simulink model "indmot1"  (Simulink 8.5)
settings: Solver=ode45  SolverMode=SingleTasking  StartTime=0.0  StopTime=3  MaxStep=1e-3  RelTol=1e-3  AbsTol=1e-6
libraries: powerlib x26
settings Model: Creator=PC  LastModifiedBy=PC
settings DataIOCC: LimitDataPoints=off
settings OptimizationCC: BlockReduction=off  BooleanDataType=off
settings DebuggingCC: SaveWithParameterizedLinksMsg=none  SignalResolutionControl=TryResolveAllWithWarning  MultiTaskDSMMsg=warning  MultiTaskCondExecSysMsg=none  FcnCallInpInsideContextMsg=UseLocalSettings
settings HardwareCC: TargetUnknown=on

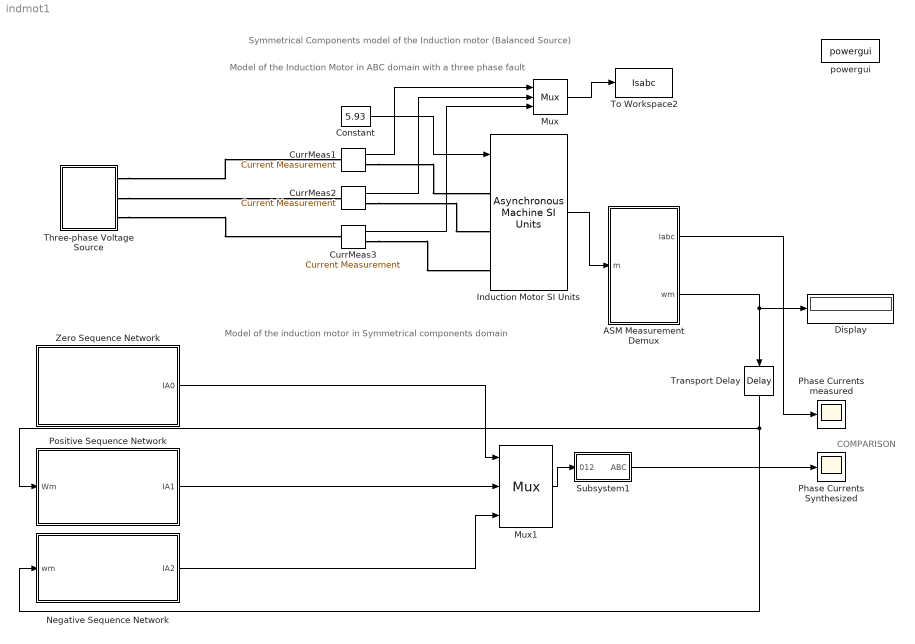
== system indmot1 ==
  note: COMPARISON
  note: Symmetrical Components model of the Induction motor (Balanced Source)
  note: Model of the Induction Motor in ABC domain with a three phase fault
  note: Model of the induction motor in Symmetrical components domain
  ASM Measurement Demux : Subsystem
  Constant : Constant  Value=5.93
  "CurrMeas1 " : powerlib/Measurements/Current Measurement  Tag=PoWeRsYsTeMmEaSuReMeNt  PhasorSimulation=off  OutputType=Complex  PSBequivalent=0
  CurrMeas2 : powerlib/Measurements/Current Measurement  Tag=PoWeRsYsTeMmEaSuReMeNt  PhasorSimulation=off  OutputType=Complex  PSBequivalent=0
  CurrMeas3 : powerlib/Measurements/Current Measurement  Tag=PoWeRsYsTeMmEaSuReMeNt  PhasorSimulation=off  OutputType=Complex  PSBequivalent=0
  Display : Display
  Induction Motor SI Units : powerlib/Machines/Asynchronous Machine SI Units  Tag=PoWeRsYsTeMbLoCk  RotorType=Squirrel-cage  PresetModel=No  MechanicalLoad=Torque Tm  ShowDetailedParameters=on  ReferenceFrame=Rotor  Units=SI  MeasurementBus=off  NominalParameters=[ 2250*746, 2400, 60 ]  Stator=[ 0.029 0.226/377]  Rotor=[ 0.022 0.226/377]  Cage1=[ 0.022 0.226/377]  Cage2=[ 0.022 0.226/377]  Lm=13.04/377  Mechanical="[ 63.87 0  2 ]"  PolePairs=2  InitialConditions=[1 0 0 0 0 0 0 0]  SimulateSaturation=off  Saturation=[14.03593122, 27.81365428, 53.79336849, 72.68890987, 97.98006896, 148.6815601, 215.7428561, 302.9841135, 428.7778367 ; 230, 322, 414, 460, 506, 552, 598, 644, 690]  LoadFlowParameters=1492000  TsPowergui=0  TsBlock=-1  IterativeModel=Forward Euler  Pmec=1.492e+006
  Mux : Mux  Inputs=3
  Mux1 : Mux  Inputs=3
  Negative Sequence Network : Subsystem
      mask Display: disp('Negative Sequence\nNetwork \nfor the\n Induction Motor')
  Phase Currents Synthesized : Scope
      settings: TickLabels=on  YMin=-75  YMax=75
  Phase Currents measured : Scope
      settings: TickLabels=on  YMin=-100  YMax=100
  Positive Sequence Network : Subsystem
      mask Display: disp('Positive Sequence\nNetwork \nfor the\n Induction Motor')
  Subsystem1 : Subsystem
  Three-phase Voltage Source : Subsystem
  To Workspace2 : ToWorkspace  VariableName=Isabc  SampleTime=-1
  Transport Delay : TransportDelay  DelayTime=1/60/360/1000
  Zero Sequence Network : Subsystem
      mask Display: disp('Zero Sequence\nNetwork \nfor the\n Induction Motor')
  powergui : powerlib/powergui  SimulationMode=Continuous  SolverType=Tustin/Backward Euler (TBE)  SampleTime=0  frequency=60  SPID=off  DisableSnubberDevices=off  DisableRonSwitches=off  DisableVfSwitches=off  SwTol=0  DisplayEquations=off  Interpol=off  methode=off  Ts=0  FunctionMessages=off  echomessages=off  HookPort=off  EnableUseOfTLC=off  x0status=blocks  frequencyindice=60  Pbase=100e6  ErrMax=1e-4  Iterations=50  UnitsV=kV  UnitsW=MW  buscounter=0  RestoreLinks=warning  ResistiveCurrentMeasurement=off  Frange=[0:2:500]  Ylog=off  Xlog=on  ShowGrid=off  save=off  variable=ZData  structure=0  ZoomFFT=on  StartTime=0.0  cycles=1  DisplayStyle=1  fundamental=60  FreqAxis=off  MaxFrequency=1000  frequencyindicesteady=1  RmsSteady=1  display=off
  wires:
  Mux/1 -> To Workspace2/1
  Mux1/1 -> Subsystem1/1(012)
  Positive Sequence Network/1(IA1) -> Mux1/2
  Negative Sequence Network/1(IA2) -> Mux1/3
  Zero Sequence Network/1(IA0) -> Mux1/1
  ASM Measurement Demux/1(Iabc) -> Phase Currents measured/1
  Subsystem1/1(ABC) -> Phase Currents Synthesized/1
  ASM Measurement Demux/2(wm) -> Display/1, Transport Delay/1
  Transport Delay/1 -> Negative Sequence Network/1(wm), Positive Sequence Network/1(Wm)
  CurrMeas2/1 -> Mux/2
  CurrMeas3/1 -> Mux/3
  "CurrMeas1 "/1 -> Mux/1
  Constant/1 -> Induction Motor SI Units/1
  Induction Motor SI Units/1 -> ASM Measurement Demux/1(m)
  connections:
  Three-phase Voltage Source/RConn1 -- "CurrMeas1 "/LConn1
  Three-phase Voltage Source/RConn2 -- CurrMeas2/LConn1
  Three-phase Voltage Source/RConn3 -- CurrMeas3/LConn1
  CurrMeas3/RConn1 -- Induction Motor SI Units/LConn3
  "CurrMeas1 "/RConn1 -- Induction Motor SI Units/LConn1
  CurrMeas2/RConn1 -- Induction Motor SI Units/LConn2

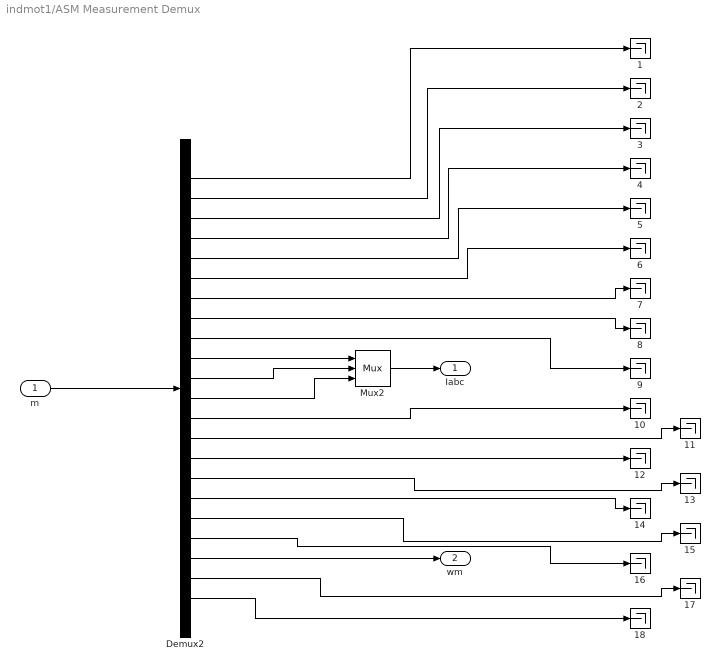
== system indmot1/ASM Measurement Demux ==
  m : Inport
  {1..18} (18 alike) : Terminator
  Demux2 : Demux  Outputs=22
  Mux2 : Mux  Inputs=3
  Iabc : Outport  InitialOutput=0
  wm : Outport  Port=2  InitialOutput=0
  wires:
  Mux2/1 -> Iabc/1
  m/1 -> Demux2/1
  Demux2/20 -> wm/1
  Demux2/10 -> Mux2/1
  Demux2/11 -> Mux2/2
  Demux2/12 -> Mux2/3
  Demux2/1 -> 1/1
  Demux2/2 -> 2/1
  Demux2/3 -> 3/1
  Demux2/4 -> 4/1
  Demux2/5 -> 5/1
  Demux2/6 -> 6/1
  Demux2/7 -> 7/1
  Demux2/8 -> 8/1
  Demux2/9 -> 9/1
  Demux2/13 -> 10/1
  Demux2/14 -> 11/1
  Demux2/15 -> 12/1
  Demux2/16 -> 13/1
  Demux2/17 -> 14/1
  Demux2/18 -> 15/1
  Demux2/19 -> 16/1
  Demux2/21 -> 17/1
  Demux2/22 -> 18/1

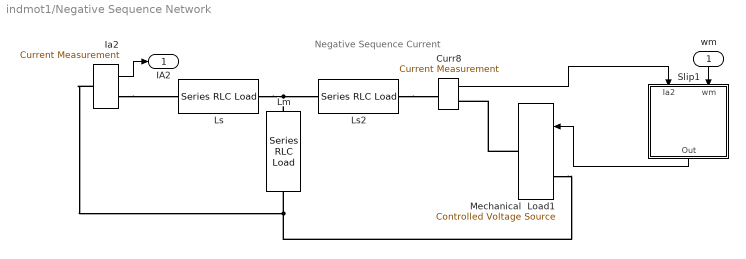
== system indmot1/Negative Sequence Network ==
  note: Negative Sequence Current
  wm : Inport
  Curr8 : powerlib/Measurements/Current Measurement  Tag=PoWeRsYsTeMmEaSuReMeNt  PhasorSimulation=off  OutputType=Complex  PSBequivalent=0
  Ia2 : powerlib/Measurements/Current Measurement  Tag=PoWeRsYsTeMmEaSuReMeNt  PhasorSimulation=off  OutputType=Complex  PSBequivalent=0
  Lm : powerlib/Elements/Series RLC Load  LConnTagsString=a  RConnTagsString=__new0  NominalVoltage=1000  NominalFrequency=60  ActivePower=10e3  InductivePower=100  CapacitivePower=100  Setx0=off  InitialVoltage=0  SetiL0=off  InitialCurrent=0  Measurements=None
  Ls : powerlib/Elements/Series RLC Load  LConnTagsString=a  RConnTagsString=__new0  NominalVoltage=1000  NominalFrequency=60  ActivePower=10e3  InductivePower=100  CapacitivePower=100  Setx0=off  InitialVoltage=0  SetiL0=off  InitialCurrent=0  Measurements=None
  Ls2 : powerlib/Elements/Series RLC Load  LConnTagsString=a  RConnTagsString=__new0  NominalVoltage=1000  NominalFrequency=60  ActivePower=10e3  InductivePower=100  CapacitivePower=100  Setx0=off  InitialVoltage=0  SetiL0=off  InitialCurrent=0  Measurements=None
  Mechanical  Load1 : powerlib/Electrical Sources/Controlled Voltage Source  Tag=PoWeRsYsTeMbLoCk  Initialize=on  Source_Type=AC  Amplitude=0  Phase=0  Frequency=0  Measurements=None
  Slip1 : Subsystem
      mask Display: disp('Calculation of:\nIa2*(Rr(s-1)/(2-s)')
  IA2 : Outport  InitialOutput=0
  wires:
  Slip1/1(Out) -> Mechanical  Load1/1
  wm/1 -> Slip1/2(wm)
  Ia2/1 -> IA2/1
  Curr8/1 -> Slip1/1(Ia2)
  connections:
  Mechanical  Load1/RConn1 -- Curr8/RConn1
  Ia2/RConn1 -- Ls/LConn1
  Ls/RConn1 -- Lm/LConn1 -- Ls2/LConn1
  Ls2/RConn1 -- Curr8/LConn1
  Ia2/LConn1 -- Mechanical  Load1/LConn1 -- Lm/RConn1

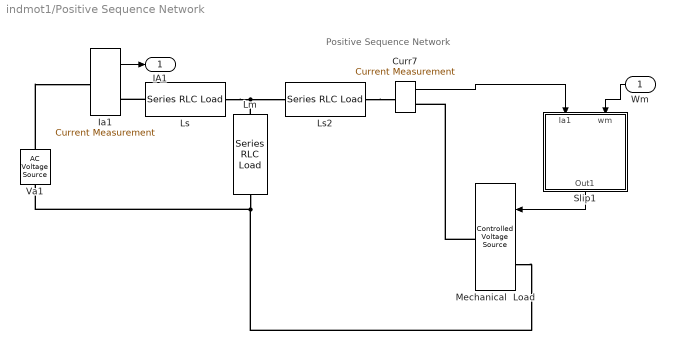
== system indmot1/Positive Sequence Network ==
  note: Positive Sequence Network
  Wm : Inport
  Curr7 : powerlib/Measurements/Current Measurement  Tag=PoWeRsYsTeMmEaSuReMeNtFiRsT  PhasorSimulation=off  OutputType=Complex  PSBequivalent=0
  Ia1 : powerlib/Measurements/Current Measurement  Tag=PoWeRsYsTeMmEaSuReMeNt  PhasorSimulation=off  OutputType=Complex  PSBequivalent=0
  Lm : powerlib/Elements/Series RLC Load  LConnTagsString=a  RConnTagsString=__new0  NominalVoltage=1000  NominalFrequency=60  ActivePower=10e3  InductivePower=100  CapacitivePower=100  Setx0=off  InitialVoltage=0  SetiL0=off  InitialCurrent=0  Measurements=None
  Ls : powerlib/Elements/Series RLC Load  LConnTagsString=a  RConnTagsString=__new0  NominalVoltage=1000  NominalFrequency=60  ActivePower=10e3  InductivePower=100  CapacitivePower=100  Setx0=off  InitialVoltage=0  SetiL0=off  InitialCurrent=0  Measurements=None
  Ls2 : powerlib/Elements/Series RLC Load  LConnTagsString=a  RConnTagsString=__new0  NominalVoltage=1000  NominalFrequency=60  ActivePower=10e3  InductivePower=100  CapacitivePower=100  Setx0=off  InitialVoltage=0  SetiL0=off  InitialCurrent=0  Measurements=None
  Mechanical  Load : powerlib/Electrical Sources/Controlled Voltage Source  Tag=PoWeRsYsTeMbLoCk  Initialize=on  Source_Type=AC  Amplitude=0  Phase=0  Frequency=0  Measurements=None
  Slip1 : Subsystem
      mask Display: disp('Calculation of:\nIa1*(Rr(1-s)/s')
  Va1 : powerlib/Electrical Sources/AC Voltage Source  Tag=PoWeRsYsTeMbLoCk  Amplitude=100  Phase=0  Frequency=60  SampleTime=0  Measurements=None
  IA1 : Outport  InitialOutput=0
  wires:
  Wm/1 -> Slip1/2(wm)
  Slip1/1(Out1) -> Mechanical  Load/1
  Ia1/1 -> IA1/1
  Curr7/1 -> Slip1/1(Ia1)
  connections:
  Mechanical  Load/RConn1 -- Curr7/RConn1
  Ls2/RConn1 -- Curr7/LConn1
  Lm/LConn1 -- Ls/RConn1 -- Ls2/LConn1
  Ls/LConn1 -- Ia1/RConn1
  Va1/RConn1 -- Ia1/LConn1
  Lm/RConn1 -- Mechanical  Load/LConn1 -- Va1/LConn1

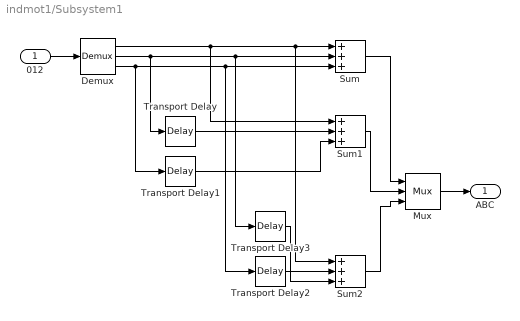
== system indmot1/Subsystem1 ==
  012 : Inport
  Demux : Demux  Outputs=3
  Mux : Mux  Inputs=3
  Sum : Sum  Inputs=+++  SaturateOnIntegerOverflow=on  InputSameDT=on  OutDataTypeStr=Inherit: Same as first input
  Sum1 : Sum  Inputs=+++  SaturateOnIntegerOverflow=on  InputSameDT=on  OutDataTypeStr=Inherit: Same as first input
  Sum2 : Sum  Inputs=+++  SaturateOnIntegerOverflow=on  InputSameDT=on  OutDataTypeStr=Inherit: Same as first input
  Transport Delay : TransportDelay  DelayTime=1/(3*60)
  Transport Delay1 : TransportDelay  DelayTime=2/(3*60)
  Transport Delay2 : TransportDelay  DelayTime=1/(3*60)
  Transport Delay3 : TransportDelay  DelayTime=2/(3*60)
  ABC : Outport  InitialOutput=0
  wires:
  012/1 -> Demux/1
  Sum1/1 -> Mux/2
  Sum/1 -> Mux/1
  Mux/1 -> ABC/1
  Sum2/1 -> Mux/3
  Demux/2 -> Transport Delay/1, Sum/2, Transport Delay3/1
  Demux/3 -> Transport Delay1/1, Sum/3, Transport Delay2/1
  Demux/1 -> Sum1/1, Sum/1, Sum2/1
  Transport Delay/1 -> Sum1/2
  Transport Delay1/1 -> Sum1/3
  Transport Delay2/1 -> Sum2/3
  Transport Delay3/1 -> Sum2/2

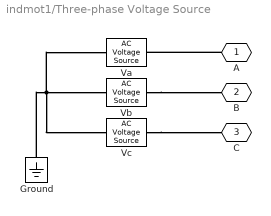
== system indmot1/Three-phase Voltage Source ==
  " Vb" : powerlib/Electrical Sources/AC Voltage Source  Tag=PoWeRsYsTeMbLoCk  Amplitude=100  Phase=0  Frequency=60  SampleTime=0  Measurements=None
  Ground : powerlib/Elements/Ground  LConnTagsString=a
  Va : powerlib/Electrical Sources/AC Voltage Source  Tag=PoWeRsYsTeMbLoCk  Amplitude=100  Phase=0  Frequency=60  SampleTime=0  Measurements=None
  Vc : powerlib/Electrical Sources/AC Voltage Source  Tag=PoWeRsYsTeMbLoCk  Amplitude=100  Phase=0  Frequency=60  SampleTime=0  Measurements=None
  A : PMIOPort  Tag=PMCPort  Port=1  Side=Right
  B : PMIOPort  Tag=PMCPort  Port=2  Side=Right
  C : PMIOPort  Tag=PMCPort  Port=3  Side=Right
  connections:
  Ground/LConn1 -- Vc/LConn1 -- " Vb"/LConn1 -- Va/LConn1
  A/RConn1 -- Va/RConn1
  " Vb"/RConn1 -- B/RConn1
  Vc/RConn1 -- C/RConn1

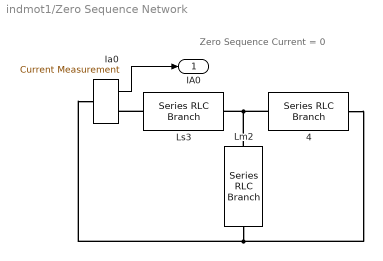
== system indmot1/Zero Sequence Network ==
  note: Zero Sequence Current = 0
  4 : powerlib/Elements/Series RLC Branch  LConnTagsString=__new0  RConnTagsString=__new0  BranchType=RLC  Resistance=1  Inductance=1e-3  SetiL0=off  InitialCurrent=0  Capacitance=1e-6  Setx0=off  InitialVoltage=0  Measurements=None
  Ia0 : powerlib/Measurements/Current Measurement  Tag=PoWeRsYsTeMmEaSuReMeNt  PhasorSimulation=off  OutputType=Complex  PSBequivalent=0
  Lm2 : powerlib/Elements/Series RLC Branch  LConnTagsString=__new0  RConnTagsString=__new0  BranchType=RLC  Resistance=1  Inductance=1e-3  SetiL0=off  InitialCurrent=0  Capacitance=1e-6  Setx0=off  InitialVoltage=0  Measurements=None
  Ls3 : powerlib/Elements/Series RLC Branch  LConnTagsString=__new0  RConnTagsString=__new0  BranchType=RLC  Resistance=1  Inductance=1e-3  SetiL0=off  InitialCurrent=0  Capacitance=1e-6  Setx0=off  InitialVoltage=0  Measurements=None
  IA0 : Outport  InitialOutput=0
  wires:
  Ia0/1 -> IA0/1
  connections:
  Lm2/RConn1 -- 4/RConn1 -- Ia0/LConn1
  Ls3/LConn1 -- Ia0/RConn1
  4/LConn1 -- Lm2/LConn1 -- Ls3/RConn1

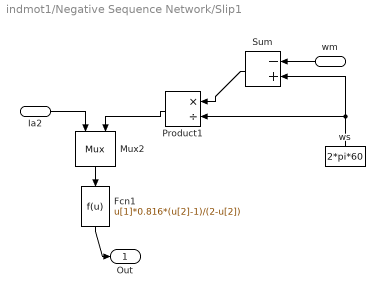
== system indmot1/Negative Sequence Network/Slip1 ==
  Ia2 : Inport
  wm : Inport  Port=2
  Fcn1 : Fcn  Expr=u[1]*0.816*(u[2]-1)/(2-u[2])
  Mux2 : Mux  Inputs=2
  Product1 : Product  Inputs=*/  SaturateOnIntegerOverflow=on  RndMeth=Zero  InputSameDT=on  OutDataTypeStr=Inherit: Same as first input
  Sum : Sum  Inputs=-+  SaturateOnIntegerOverflow=on  InputSameDT=on  OutDataTypeStr=Inherit: Same as first input
  ws : Constant  Value=2*pi*60
  Out : Outport
  wires:
  Sum/1 -> Product1/1
  Ia2/1 -> Mux2/1
  Fcn1/1 -> Out/1
  wm/1 -> Sum/1
  ws/1 -> Product1/2, Sum/2
  Product1/1 -> Mux2/2
  Mux2/1 -> Fcn1/1

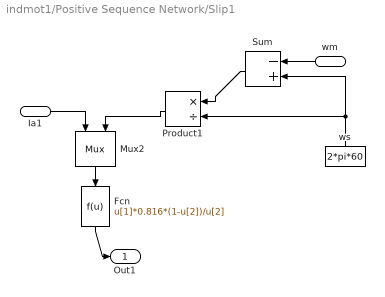
== system indmot1/Positive Sequence Network/Slip1 ==
  Ia1 : Inport
  wm : Inport  Port=2
  Fcn : Fcn  Expr=u[1]*0.816*(1-u[2])/u[2]
  Mux2 : Mux  Inputs=2
  Product1 : Product  Inputs=*/  SaturateOnIntegerOverflow=on  RndMeth=Zero  InputSameDT=on  OutDataTypeStr=Inherit: Same as first input
  Sum : Sum  Inputs=-+  SaturateOnIntegerOverflow=on  InputSameDT=on  OutDataTypeStr=Inherit: Same as first input
  ws : Constant  Value=2*pi*60
  Out1 : Outport
  wires:
  Mux2/1 -> Fcn/1
  ws/1 -> Sum/2, Product1/2
  wm/1 -> Sum/1
  Fcn/1 -> Out1/1
  Ia1/1 -> Mux2/1
  Sum/1 -> Product1/1
  Product1/1 -> Mux2/2
